simulink model "z4_regulator_symulacja"  (R2021a)
settings: Solver=VariableStepAuto  StartTime=0.0  StopTime=1.5  RelTol=1e-3
values from neighbouring files (symbols this model uses):
  sb = -8    [z4.m]    (also in z6i7.m = -5; z_dod.m = -2)
settings Model: Creator=48604  LastModifiedBy=48604

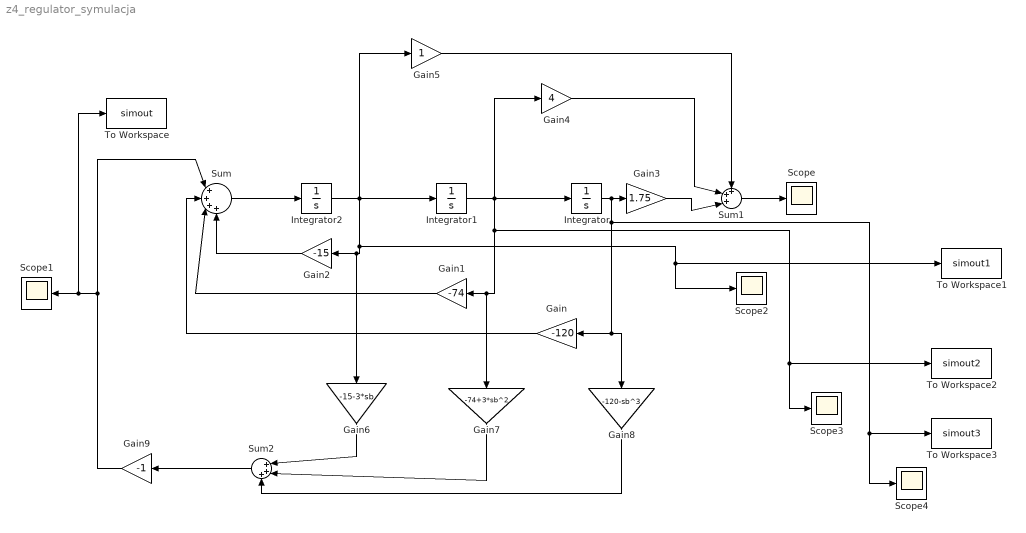
== system z4_regulator_symulacja ==
  Gain : Gain  Gain=-120
  Gain1 : Gain  Gain=-74
  Gain2 : Gain  Gain=-15
  Gain3 : Gain  Gain=1.75
  Gain4 : Gain  Gain=4
  Gain5 : Gain
  Gain6 : Gain  Gain=-15-3*sb
  Gain7 : Gain  Gain=-74+3*sb^2
  Gain8 : Gain  Gain=-120-sb^3
  Gain9 : Gain  Gain=-1
  Integrator : Integrator  InitialCondition=1
  Integrator1 : Integrator  InitialCondition=2
  Integrator2 : Integrator  InitialCondition=-1
  Scope{,1..4} (5 alike) : Scope
  Sum : Sum  Inputs=|++++
  Sum1 : Sum  Inputs=+++|
  Sum2 : Sum  Inputs=|+++
  To Workspace : ToWorkspace  VariableName=simout  SaveFormat=Structure With Time  SampleTime=-1
  To Workspace1 : ToWorkspace  VariableName=simout1  SaveFormat=Structure With Time  SampleTime=-1
  To Workspace2 : ToWorkspace  VariableName=simout2  SaveFormat=Structure With Time  SampleTime=-1
  To Workspace3 : ToWorkspace  VariableName=simout3  SaveFormat=Structure With Time  SampleTime=-1
  wires:
  Gain1/1 -> Sum/3
  Integrator1/1 -> To Workspace2/1, Scope3/1, Gain7/1, Gain1/1, Gain4/1, Integrator/1
  Gain5/1 -> Sum1/1
  Sum/1 -> Integrator2/1
  Integrator2/1 -> Scope2/1, To Workspace1/1, Gain2/1, Gain6/1, Gain5/1, Integrator1/1
  Gain2/1 -> Sum/4
  Gain3/1 -> Sum1/3
  Integrator/1 -> To Workspace3/1, Scope4/1, Gain8/1, Gain/1, Gain3/1
  Gain4/1 -> Sum1/2
  Gain/1 -> Sum/2
  Sum1/1 -> Scope/1
  Gain9/1 -> To Workspace/1, Scope1/1, Sum/1
  Gain6/1 -> Sum2/1
  Gain7/1 -> Sum2/2
  Gain8/1 -> Sum2/3
  Sum2/1 -> Gain9/1
